simulink model "gmm_sim"  (R2013b)
settings: Solver=ode1  SolverMode=SingleTasking  StartTime=0.0  StopTime=60  FixedStep=0.01  MaxStep=0.01  RelTol=1e-3  AbsTol=1e-6
settings Model: ExtModeTrigMode=oneshot  ExtModeArmWhenConnect=off  Creator=MK  LastModifiedBy=MK
settings SolverCC: InitialStep=0.01
settings DataIOCC: Decimation=100  MaxDataPoints=61  SignalLoggingSaveFormat=ModelDataLogs
settings OptimizationCC: BlockReduction=off  BooleanDataType=off
settings DebuggingCC: SaveWithParameterizedLinksMsg=none  SignalResolutionControl=TryResolveAllWithWarning  SolverPrmCheckMsg=none  MultiTaskDSMMsg=warning  MultiTaskCondExecSysMsg=none
settings HardwareCC: TargetUnknown=on
settings RTWCC: TemplateMakefile=grt_vc.tmf  IncludeERTFirstTime=on
settings GRTTargetCC: CombineOutputUpdateFcns=off  GRTInterface=on

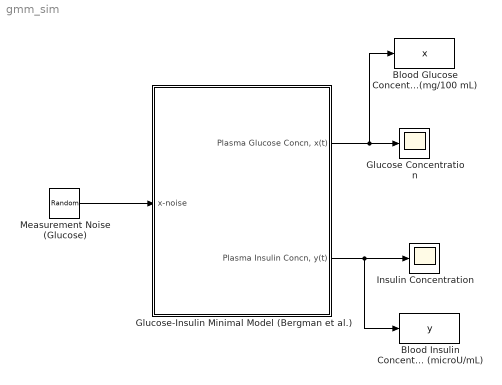
== system gmm_sim ==
  Blood Glucose Concentration (mg/100 mL) : ToWorkspace  VariableName=x  SampleTime=-1
      settings: Decimation=100
  Blood Insulin Concentration (microU/mL) : ToWorkspace  VariableName=y  SampleTime=-1
      settings: Decimation=100
  Glucose Concentration : Scope
      settings: TickLabels=on  TimeRange=60  YMin=0  YMax=300  MaxDataPoints=60  Decimation=100
  Glucose-Insulin Minimal Model (Bergman et al.) : Subsystem
  Insulin Concentration : Scope
      settings: TickLabels=on  TimeRange=60  YMin=-20  YMax=80  MaxDataPoints=60  Decimation=100
  Measurement Noise (Glucose) : RandomNumber  Variance=25  Seed=37  SampleTime=0
  wires:
  Measurement Noise (Glucose)/1 -> Glucose-Insulin Minimal Model (Bergman et al.)/1(x-noise)
  Glucose-Insulin Minimal Model (Bergman et al.)/1("Plasma Glucose Concn, x(t)") -> Glucose Concentration/1, Blood Glucose Concentration (mg/100 mL)/1
  Glucose-Insulin Minimal Model (Bergman et al.)/2("Plasma Insulin Concn, y(t)") -> Insulin Concentration/1, Blood Insulin Concentration (microU/mL)/1

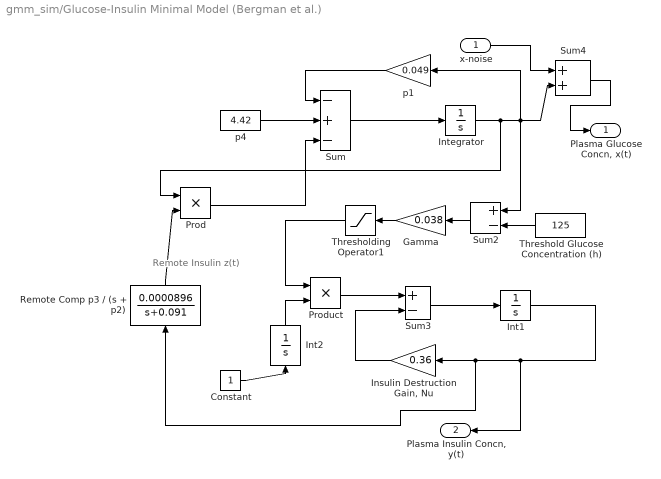
== system gmm_sim/Glucose-Insulin Minimal Model (Bergman et al.) ==
  note: Remote
      | Insulin
      | z(t)
  x-noise : Inport
  Constant : Constant
  Gamma : Gain  Gain=0.038  SaturateOnIntegerOverflow=on  OutDataTypeStr=Inherit: Same as input  ParamDataTypeStr=Inherit: Same as input
  "Insulin Destruction Gain, Nu" : Gain  Gain=0.36  SaturateOnIntegerOverflow=on  OutDataTypeStr=Inherit: Same as input  ParamDataTypeStr=Inherit: Same as input
  Int1 : Integrator  InitialCondition=76
  Int2 : Integrator  InitialCondition=0.0
  Integrator : Integrator  InitialCondition=260
  Prod : Product  SaturateOnIntegerOverflow=on  RndMeth=Zero  InputSameDT=on  OutDataTypeStr=Inherit: Same as first input
  Product : Product  SaturateOnIntegerOverflow=on  RndMeth=Zero  InputSameDT=on  OutDataTypeStr=Inherit: Same as first input
  Remote Comp p3 / (s + p2) : TransferFcn  Numerator=0.0000896  Denominator=[1 0.091]
  Sum : Sum  Inputs=-+-  SaturateOnIntegerOverflow=on  InputSameDT=on  OutDataTypeStr=Inherit: Same as first input
  Sum2 : Sum  Inputs=+-  SaturateOnIntegerOverflow=on  InputSameDT=on  OutDataTypeStr=Inherit: Same as first input
  Sum3 : Sum  Inputs=+-  SaturateOnIntegerOverflow=on  InputSameDT=on  OutDataTypeStr=Inherit: Same as first input
  Sum4 : Sum  SaturateOnIntegerOverflow=on  InputSameDT=on  OutDataTypeStr=Inherit: Same as first input
  Threshold Glucose Concentration (h) : Constant  Value=125
  Thresholding Operator1 : Saturate  UpperLimit=100000  LowerLimit=0
  p1 : Gain  Gain=0.049  SaturateOnIntegerOverflow=on  OutDataTypeStr=Inherit: Same as input  ParamDataTypeStr=Inherit: Same as input
  p4 : Constant  Value=4.42
  "Plasma Glucose Concn, x(t)" : Outport
  "Plasma Insulin Concn, y(t)" : Outport  Port=2
  wires:
  x-noise/1 -> Sum4/1
  Sum4/1 -> "Plasma Glucose Concn, x(t)"/1
  p4/1 -> Sum/2
  Thresholding Operator1/1 -> Product/1
  Int2/1 -> Product/2
  Product/1 -> Sum3/1
  Constant/1 -> Int2/1
  p1/1 -> Sum/1
  Threshold Glucose Concentration (h)/1 -> Sum2/2
  Sum2/1 -> Gamma/1
  Gamma/1 -> Thresholding Operator1/1
  "Insulin Destruction Gain, Nu"/1 -> Sum3/2
  Integrator/1 -> Sum4/2, p1/1, Sum2/1, Prod/1
  Sum3/1 -> Int1/1
  Remote Comp p3 / (s + p2)/1 -> Prod/2
  Prod/1 -> Sum/3
  Sum/1 -> Integrator/1
  Int1/1 -> Remote Comp p3 / (s + p2)/1, "Insulin Destruction Gain, Nu"/1, "Plasma Insulin Concn, y(t)"/1
